simulink model "Spectrum_Viewer"  (R2020a)
settings: Solver=VariableStepAuto  StartTime=0.0  StopTime=10.0  RelTol=1e-3
settings Model: Creator=dinhm  LastModifiedBy=dinhm

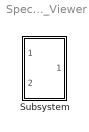
== system Spectrum_Viewer ==
  Subsystem : Subsystem

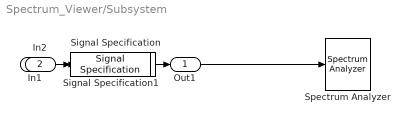
== system Spectrum_Viewer/Subsystem ==
  In1 : Inport
  In2 : Inport  Port=2
  Signal Specification : SignalSpecification  SampleTime=1/16e4
  Signal Specification1 : SignalSpecification  SampleTime=1/16e4
  Spectrum Analyzer : SpectrumAnalyzer
  Out1 : Outport
  wires:
  Signal Specification/1 -> Spectrum Analyzer/1
  In2/1 -> Signal Specification/1
  In1/1 -> Signal Specification1/1
  Signal Specification1/1 -> Out1/1
